simulink subsystem "PrimitiveBattery_refsub"  (R2026a)
settings: Solver=VariableStepAuto
libraries: fl_lib x3
settings Model: Creator=isaacito  LastModifiedBy=isaacito
settings SimscapeCC: SimscapeNominalValues="[{\"value\":\"1\",\"unit\":\"A\"},{\"value\":\"1\",\"unit\":\"bar\"},{\"value\":\"1\",\"unit\":\"cm^2\"},{\"value\":\"1\",\"unit\":\"cm^3/s\"},{\"value\":\"1\",\"unit\":\"kJ/kg\"},{\"value\":\"1\",\"unit\":\"kW\"},{\"value\":\"1\",\"unit\":\"l\"},{\"value\":\"1\",\"unit\":\"N\"},{\"value\":\"1\",\"unit\":\"N*m\"},{\"value\":\"1\",\"unit\":\"V\"}]"  SimscapeLogType=none  SimscapeLogDataHistory=5000.0

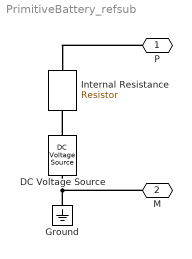
== system PrimitiveBattery_refsub ==
  DC Voltage Source : fl_lib/Electrical/Electrical Sources/DC Voltage Source  v0=340 V
      settings: AttributesFormatString=%<v0> [%<v0_unit>]
  Ground : fl_lib/Electrical/Electrical Elements/Electrical Reference
  Internal Resistance : fl_lib/Electrical/Electrical Elements/Resistor  R=0.01 Ohm  i_specify=off  i_priority=High  i=0 A  i_nominal_specify=off  i_nominal_value=1  i_nominal_unit=A  v_specify=off  v_priority=High  v=0 V  v_nominal_specify=off  v_nominal_value=1  v_nominal_unit=V
      settings: AttributesFormatString=%<R> [%<R_unit>]
  P : PMIOPort  Side=Right
  M : PMIOPort  Port=2  Side=Right
  connections:
  DC Voltage Source/RConn1 -- Ground/LConn1 -- M/RConn1
  P/RConn1 -- Internal Resistance/RConn1
  DC Voltage Source/LConn1 -- Internal Resistance/LConn1
